simulink model "bpsk"  (R2012b)
settings: Solver=ode45  StartTime=0.0  StopTime=50  RelTol=1e-3
undefined symbols (not defined in the file or in its folder): DiscIntNeverNeededParam
libraries: commfilt2 x4, dspsigops x2, commseqgen2 x1
settings Model: Creator=Matt  LastModifiedBy=Matt

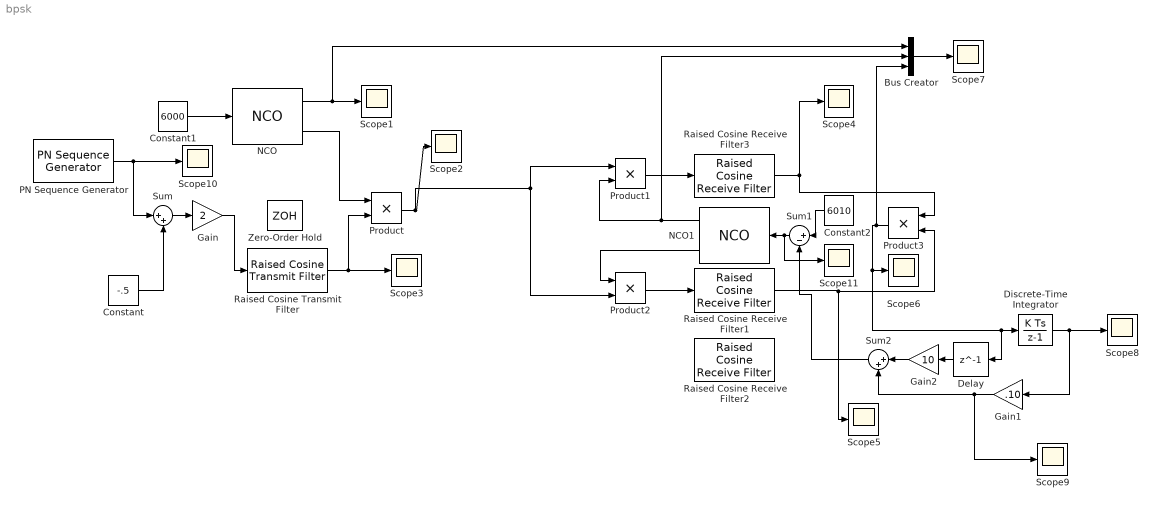
== system bpsk ==
  Bus Creator : BusCreator  Inputs=3
  Constant : Constant  Value=-.5
  Constant1 : Constant  Value=6000  OutDataTypeStr=int32
  Constant2 : Constant  Value=6010  OutDataTypeStr=int32
  Delay : Delay  DelayLength=1
  Discrete-Time Integrator : DiscreteIntegrator  gainval=1  SampleTime=-1  OutDataTypeStr=double  ICPrevOutput=DiscIntNeverNeededParam  ICPrevScaledInput=DiscIntNeverNeededParam
  Gain : Gain  Gain=2
  Gain1 : Gain  Gain=.10  OutDataTypeStr=int32
  Gain2 : Gain  Gain=10  OutDataTypeStr=int32
  NCO : dspsigops/NCO  AccIncSrc=Input port  AccInc=100  PhaseOffsetSrc=Specify via dialog  PhaseOffset=0  AccumWL=16  HasDither=on  DitherWL=4  PNgeneratorLength=19  HasPhaseQuantizer=on  TableDepth=12  HasOutputPhaseError=off  Formula=Sine and cosine  DataType=double  OutputWL=16  OutputFL=14  CompMethod=Table lookup (no interpolation)  SampleTime=1  SamplesPerFrame=1
  NCO1 : dspsigops/NCO  AccIncSrc=Input port  AccInc=100  PhaseOffsetSrc=Specify via dialog  PhaseOffset=0  AccumWL=16  HasDither=on  DitherWL=4  PNgeneratorLength=19  HasPhaseQuantizer=on  TableDepth=12  HasOutputPhaseError=off  Formula=Sine and cosine  DataType=double  OutputWL=16  OutputFL=14  CompMethod=Table lookup (no interpolation)  SampleTime=1  SamplesPerFrame=1
  PN Sequence Generator : commseqgen2/PN Sequence Generator  poly=[1 0 0 0 0 1 1]  ini_sta=[0 0 0 0 0 1]  outBitMaskSource=Dialog parameter  shift=0  outVarSiz=off  maxOutSizeMode=Dialog parameter  maxOutSize=[10 1]  Ts=.1  frameBased=off  sampPerFrame=1  reset=off  bitPackedOutputs=off  outDataType=double  numPackedBits=8  bitPackDataSigned=off  bitPackedOutDType=double
  Product{,1..3} (4 alike) : Product  RndMeth=Zero
  Raised Cosine Receive Filter1 : commfilt2/Raised Cosine Receive Filter  filtType=Square root  N=100  D=5  R=0.2  sampMode=Mute  saveAsFlag=0  rateMode=None  downFactor=8  downOffset=0  framing=Allow multirate processing  checkGain=Normalized  filterGain=1  checkCoeff=off  variableName=rcRxFilt1  launchFVT=off  roundingMode=Floor  overflowMode=off
  Raised Cosine Receive Filter2 : commfilt2/Raised Cosine Receive Filter  filtType=Square root  N=100  D=5  R=0.2  sampMode=Mute  saveAsFlag=0  rateMode=None  downFactor=8  downOffset=0  framing=Allow multirate processing  checkGain=Normalized  filterGain=1  checkCoeff=off  variableName=rcRxFilt2  launchFVT=off  roundingMode=Floor  overflowMode=off
  Raised Cosine Receive Filter3 : commfilt2/Raised Cosine Receive Filter  filtType=Square root  N=100  D=5  R=0.2  sampMode=Mute  saveAsFlag=0  rateMode=None  downFactor=8  downOffset=0  framing=Allow multirate processing  checkGain=Normalized  filterGain=1  checkCoeff=off  variableName=rcRxFilt3  launchFVT=off  roundingMode=Floor  overflowMode=off
  Raised Cosine Transmit Filter : commfilt2/Raised Cosine Transmit Filter  filtType=Square root  D=5  R=0.2  sampMode=Mute  saveAsFlag=0  N=100  framing=Allow multirate processing  InputProcessing=Columns as channels (frame based)  checkGain=Normalized  filterGain=1  checkCoeff=off  variableName=rcTxFilt  launchFVT=off  roundingMode=Floor  overflowMode=off
  Scope{1..11} (11 alike) : Scope
      Scope10 settings: YMin=-0.4  YMax=0.2  SaveName=ScopeData9
      Scope11 settings: YMin=5920  YMax=5952.5  SaveName=ScopeData10
      Scope3 settings: YMin=-0.15  YMax=0.15  SaveName=ScopeData2
      Scope4 settings: YMin=-0.25  YMax=0.3  SaveName=ScopeData3
      Scope5 settings: SaveName=ScopeData4
      Scope6 settings: SaveName=ScopeData5
      Scope7 settings: SaveName=ScopeData6
      Scope8 settings: SaveName=ScopeData7
      Scope9 settings: SaveName=ScopeData8
  Sum : Sum  Inputs=|++
  Sum1 : Sum  Inputs=|+-
  Sum2 : Sum  Inputs=|++
  Zero-Order Hold : ZeroOrderHold  SampleTime=.001
  wires:
  Sum/1 -> Gain/1
  Constant/1 -> Sum/2
  Constant1/1 -> NCO/1
  NCO/1 -> Bus Creator/1, Scope1/1
  NCO/2 -> Product/1
  Product/1 -> Product1/1, Product2/2, Scope2/1
  NCO1/1 -> Bus Creator/2, Product1/2
  NCO1/2 -> Product2/1
  Product1/1 -> Raised Cosine Receive Filter3/1
  Raised Cosine Receive Filter3/1 -> Scope4/1, Product3/1
  Product2/1 -> Raised Cosine Receive Filter1/1
  Raised Cosine Receive Filter1/1 -> Product3/2, Scope5/1
  Product3/1 -> Bus Creator/3, Delay/1, Discrete-Time Integrator/1, Scope6/1
  Bus Creator/1 -> Scope7/1
  Discrete-Time Integrator/1 -> Gain1/1, Scope8/1
  Sum1/1 -> Scope11/1, NCO1/1
  Constant2/1 -> Sum1/1
  PN Sequence Generator/1 -> Scope10/1, Sum/1
  Gain/1 -> Raised Cosine Transmit Filter/1
  Sum2/1 -> Sum1/2
  Gain2/1 -> Sum2/1
  Gain1/1 -> Scope9/1, Sum2/2
  Delay/1 -> Gain2/1
  Raised Cosine Transmit Filter/1 -> Scope3/1, Product/2
